simulink model "motorPosition"  (R2020a)
settings: Solver=VariableStepAuto  StartTime=0.0  StopTime=10.0  RelTol=1e-3
values from neighbouring files (symbols this model uses):
  b = 3.5077E-6    [motor_parameter.sldd]
  J = 3.3384E-6    [motor_parameter.sldd]
  K = 0.0274    [motor_parameter.sldd]
  L = 2.75E-6    [motor_parameter.sldd]
  R = 4.0    [motor_parameter.sldd]
settings Model: DataDictionary=motor_parameter.sldd  Creator=INDRAJIT MARATHE  LastModifiedBy=INDRAJIT MARATHE
settings DataIOCC: SaveOutput=off  SaveTime=off

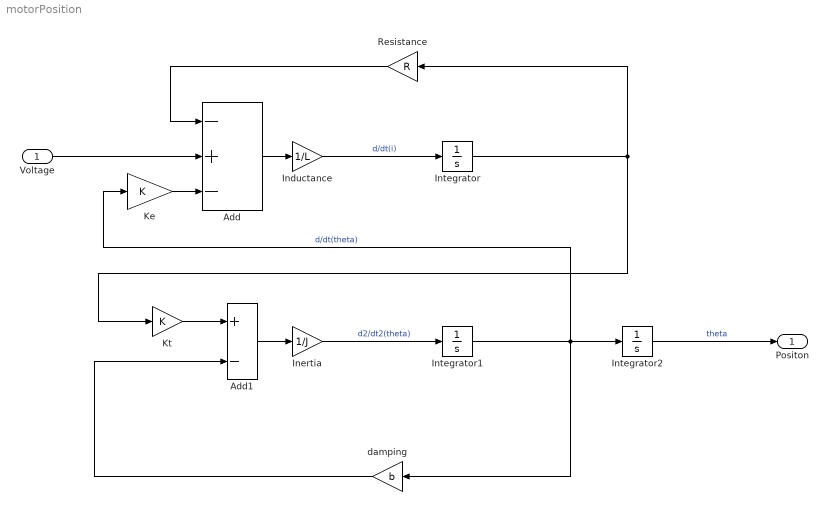
== system motorPosition ==
  Voltage : Inport  OutDataTypeStr=double  PortDimensions=1  SampleTime=0
  " Add" : Sum  Inputs=-+-
  " Add1" : Sum  Inputs=+-
  " Integrator" : Integrator
  " Integrator1" : Integrator
  " Integrator2" : Integrator
  Inductance : Gain  Gain=1/L
  Inertia : Gain  Gain=1/J
  Ke : Gain  Gain=K
  Kt : Gain  Gain=K
  Resistance : Gain  Gain=R
  damping : Gain  Gain=b
  " Positon" : Outport  OutDataTypeStr=double  PortDimensions=1  SampleTime=0
  wires:
  " Integrator1"/1 -> " Integrator2"/1, damping/1, Ke/1  "d/dt(theta)"
  damping/1 -> " Add1"/2
  " Integrator"/1 -> Resistance/1, Kt/1
  " Add"/1 -> Inductance/1
  Inductance/1 -> " Integrator"/1  "d/dt(i)"
  " Add1"/1 -> Inertia/1
  Voltage/1 -> " Add"/2
  Kt/1 -> " Add1"/1
  " Integrator2"/1 -> " Positon"/1  "theta"
  Resistance/1 -> " Add"/1
  Ke/1 -> " Add"/3
  Inertia/1 -> " Integrator1"/1  "d2/dt2(theta)"
